simulink model "PAMsystem"  (Simulink 7.7)
settings: Solver=FixedStepDiscrete  StartTime=0.0  StopTime=1  RelTol=1e-3
values from neighbouring files (symbols this model uses):
  D = [  1 -1  1 -1  1  1 -1 -1 ... (first row only)    [cdma.m]    (also in compressed_sampling.m = idct(eye(5000,5000)))
libraries: commchan3 x1, commsink2 x1, commrandsrc2 x1, dspsigops x1
settings Model: Creator=ArunKB  LastModifiedBy=ArunKB

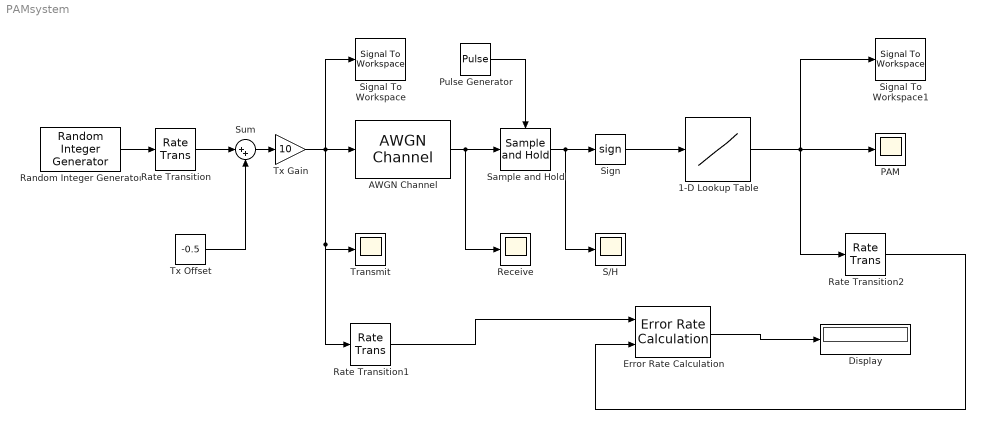
== system PAMsystem ==
  1-D Lookup Table : Lookup_n-D  NumberOfTableDimensions=1  BreakpointsForDimension1=[-1,0,1]  Table=[-5,-5,5]  RndMeth=Simplest  InputSameDT=on
  AWGN Channel : commchan3/AWGN Channel  SystemSampleTime=-1  InputProcessing=Columns as channels (frame based)  seed=randseed  noiseMode=Variance from mask  EbNodB=10  EsNodB=10  SNRdB=10  bitsPerSym=1  Ps=1  Tsym=1  variance=5.5
  Display : Display
  Error Rate Calculation : commsink2/Error Rate Calculation  N=1  st_delay=0  cp_mode=Entire frame  subframe=[]  PMode=Port  WsName=ErrorVec  RsMode2=off  stop=off  numErr=100  maxBits=1e6
  PAM : Scope
      settings: SaveName=PAM  DataFormat=Array
  Pulse Generator : DiscretePulseGenerator  PulseType=Time based  Period=(1e-3)/2  PulseWidth=5  PhaseDelay=(1e-3)/2
  Random Integer Generator : commrandsrc2/Random Integer Generator  SystemSampleTime=-1  mul=2  seed=randseed  Ts=1e-3  frameBased=off  sampPerFrame=1  orient=on  outDataType=double
  Rate Transition : RateTransition
  Rate Transition1 : RateTransition
  Rate Transition2 : RateTransition
  Receive : Scope
  S/H : Scope
      settings: SaveName=ScopeData3
  Sample and Hold : dspsigops/Sample and Hold  SystemSampleTime=-1  trig=Rising edge  initCond=0  latchinput=off
  Sign : Signum
  Signal To Workspace : SignalToWorkspace  VariableName=Transmit  SaveFormat=Array  Save2DMode=2-D array (concatenate along first dimension)
      settings: CopyFcn=dspblkcopystw(gcbh);
  Signal To Workspace1 : SignalToWorkspace  VariableName=PAM  SaveFormat=Array  Save2DMode=2-D array (concatenate along first dimension)
      settings: CopyFcn=dspblkcopystw(gcbh);
  Sum : Sum  Inputs=|++
  Transmit : Scope
      settings: SaveName=Transmit  DataFormat=Array
  Tx Gain : Gain  Gain=10
  Tx Offset : Constant  Value=-0.5
  wires:
  Tx Offset/1 -> Sum/2
  Sample and Hold/1 -> Sign/1, S/H/1
  Random Integer Generator/1 -> Rate Transition/1
  Rate Transition/1 -> Sum/1
  Sum/1 -> Tx Gain/1
  Tx Gain/1 -> AWGN Channel/1, Signal To Workspace/1, Transmit/1, Rate Transition1/1
  AWGN Channel/1 -> Sample and Hold/1, Receive/1
  Sign/1 -> 1-D Lookup Table/1
  1-D Lookup Table/1 -> PAM/1, Signal To Workspace1/1, Rate Transition2/1
  Pulse Generator/1 -> Sample and Hold/Trigger
  Rate Transition2/1 -> Error Rate Calculation/2
  Rate Transition1/1 -> Error Rate Calculation/1
  Error Rate Calculation/1 -> Display/1
